simulink model "Sim_normboundsystem_iqctest"  (Simulink 7.3)
settings: Solver=ode45  StartTime=0.0  StopTime=10  RelTol=1e-3
settings Model: Creator=MD710  LastModifiedBy=MD710
settings DebuggingCC: SaveWithParameterizedLinksMsg=none  SolverPrmCheckMsg=none  MultiTaskDSMMsg=warning  MultiTaskCondExecSysMsg=none  FcnCallInpInsideContextMsg=Enable All  StrictBusMsg=None
settings HardwareCC: TargetHWDeviceType=32-bit Generic
settings RTWCC: IncludeERTFirstTime=on
settings GRTTargetCC: TargetFcnLib=ansi_tfl_tmw.mat

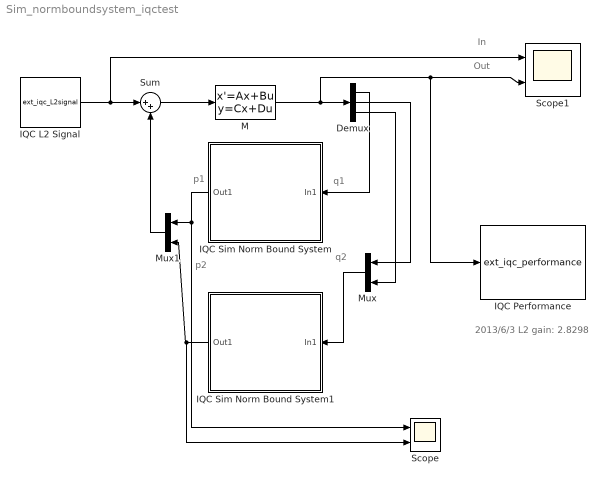
== system Sim_normboundsystem_iqctest ==
  note: p1
  note: q1
  note: q2
  note: p2
  note: 2013/6/3 L2 gain: 2.8298
  note: In
  note: Out
  Demux : Demux  Outputs=3
  IQC L2 Signal : M-S-Function  FunctionName=ext_iqc_L2signal  Parameters=sig_size,sam_time,sig_type,tru_time,sig_amp,sig_fre,user_cus  mask(IQC L2 signal(ver:0.1)){sig_size=2, sam_time=0, sig_type=Sine wave, tru_time=5, sig_amp=1, sig_fre=2, user_cus='2*exp(3*t)'}
      mask prompts: sig_size "Signal Dimension:(Default: 1)"; sam_time "Sample Time:(Default: 0)"; sig_type "Signal Type:"; tru_time "Truncation Time:"; sig_amp "Maximum Amplitude:"; sig_fre "Frequency:"; user_cus "Custom:"
      mask help:
      | Important:
      | In IQC procedure step (as commond iqc_gain_tbx, the task is get
      | L2 gain value), regardless of the user to choose which option (ex sine...),
      | here regarded as generalized L2 signal.
      mask StyleString: edit,edit,popup(Step|Square wave|Sine wave|Custom|Random|External),edit,edit,edit,edit
      mask CallbackString: ||iqc_block_cho(gcb,'L2signal_type')||||
      mask TabNameString: Main,Main,Simulation,Simulation,Simulation,Simulation,Simulation
      mask Display: plot(0:0.1:10,[sin(0:0.1:6.2) zeros(1,38)])
  IQC Performance : M-S-Function  FunctionName=ext_iqc_performance  Parameters=imp_met,save_lin_com,isiqcbode,fre_ran,uselmitool,lmi_par  mask(IQC Performance(ver:0.1)){imp_met=Calculation and Simulation, save_lin_com=off, isiqcbode=off, fre_ran='', uselmitool=lmilab, lmi_par=''}
      mask prompts: imp_met "Implementation Methods"; save_lin_com "Save the Linear File and Command File"; isiqcbode "Display IQC Bode Figure"; fre_ran "Frequency Range:(Default: empty)"; uselmitool "LMI Tool:"; lmi_par "Parameter:(if empty use define)"
      mask help:
      | Important:
      | In IQC toolbox calculate step (as commond iqc_gain_tbx, the task is get
      | L2 gain value), regardless of the user to connect any signal input(Even if
      | not a signal), here regarded as generalized L2 signal.
      |
      | Example 1: setlmioptions('',[0 200 0 0 777])
      | the block parameter is
      | LMI Tool: lmilab
      | Parameter:
      |        [0 200 0 0 777]
      |
      | Example 2: setlmioptions('yalmip','solver','sdpt3','verbose',1)
      | the block parameter is
      | LMI Tool: yalmip
      | Parameter:
      |        {'solver',sdpt3','verbose',1}
      mask Help:
      | <a href="matlab:doc abst_init_iqc;">abst_init_iqc</a>
      | <a href="matlab:doc setlmioptions;">setlmioptions</a>
      | <a href="matlab:doc iqc_gain_tbx;">iqc_gain_tbx</a>
      mask StyleString: popup(Calculation and Simulation|Only Calculation|Only Simulation),checkbox,checkbox,edit,popup(lmilab|yalmip),edit
      mask CallbackString: iqc_block_cho(gcb,'performance_imp')||iqc_block_cho(gcb,'performance_bodefre')|||
      mask TabNameString: Main,Main,Main,Main,LMI,LMI
      mask Display: fprintf('In -> Out \n performance \n L2 gain:\n%4.4f',2.8297);
  IQC Sim Norm Bound System : Subsystem  mask(IQC Sim Norm Bound System(ver:0.1)){sou_sys=Random, num_inp=1, num_out=1, num_sta=3, upp_bou=1, sam_tim=0, cus='1/(s+1)', var_nam='', iqc1=on, iqc1_pole=[4], iqc1_out='', iqc2=on, lis_rel='out==iqc_ltigain(in)', swsystemtype=0, A=0, B=0, C=0, D=0, newsam_tim=0}
      mask prompts: sou_sys "Source of the system:(Default: Random)"; num_inp "The Number of Input:(Default: 1)"; num_out "The Number of Output:(Default: 1)"; num_sta "The Number of States:(Default: 1)"; upp_bou "Upper Bound of the Hinf-Norm:(default: 1)"; sam_tim "Sample Time:(Default: 0)"; cus "Custom: (Default: '1/(s+1)' or '1/(z+0.5)')"; var_nam "Variable Name:(Default: empty)"; iqc1 "iqc_ltiunmod(Input,Pole,Number Output,Upper Bound)"; iqc1_pole "Pole:(Default: [1])"; iqc1_out "Output Variable:(Default: empty)"; iqc2 "Custom IQC"; lis_rel "List of IQC Relationships:"; newsam_tim "Mask Parameter 19:"
      mask init:
      | swsystemtype=1;
      | A=randn(num_sta);
      | B=randn(num_sta,num_inp);
      | C=randn(num_out,num_sta);
      | D=randn(num_out,num_inp);
      | switch sou_sys
      |     case 1
      |         if sam_tim==0
      |             newsam_tim=1;
      |             A=A-(1+max(real(eig(A))))*eye(num_sta);
      |             G=ss(A,B,C,D);
      |             normG=norm(G,inf);
      |             G=G*upp_bou*rand/normG;
      |         elseif sam_tim>0
      |             newsam_tim=sam_tim;
      |             swsystemtype=2;
      |             A=A-(1+max(real(eig(A))))*eye(num_sta);
      |             G=ss(A,B,C,D);
      |             normG=norm(G,inf);
      |             G=G*upp_bou*rand/normG;
      |             G=c2d(G,sam_tim);
      |         else
      |             error(['sampletime set error'])
      |         end
      |     case 2
      |         s=tf('s');
      |         newsam_tim=1;
      |         if sam_tim>0
      |             newsam_tim=sam_tim;
      |             swsystemtype=2;
      |             z=tf('z',sam_tim);
      |         end
      |         if ischar(cus)
      |             eval(['G=ss(',cus,');']);
      |         else
      |             G=ss(cus);
      |         end
      | end
      | A=G.a;
      | B=G.b;
      | C=G.c;
      | D=G.d;
      mask Help: <a href="matlab:doc iqc_ltiunmod;">iqc_ltiunmod</a>
      mask StyleString: popup(Random|Custom),edit,edit,edit,edit,edit,edit,edit,checkbox,edit,edit,checkbox,edit,edit,edit,edit,edit,edit,edit
      mask CallbackString: iqc_block_cho(gcb,'sim_normboundsys_sou')||||||||iqc_block_cho(gcb,'sim_normboundsys_iqc1')|||iqc_block_cho(gcb,'sim_normboundsys_iqc2')|||||||
      mask TabNameString: Simulink Parameters,Simulink Parameters,Simulink Parameters,Simulink Parameters,Simulink Parameters,Simulink Parameters,Simulink Parameters,Simulink Parameters,Procedure Parameters,Procedure Parameters,Procedure Parameters,Procedure Parameters,Procedure Parameters,Simulink Parameters,Simulink Parameters,Simulink Parameters,Simulink Parameters,Simulink Parameters,Simulink Parameters
      mask Display: disp('\fontsize{14}||\Delta|| < k', 'texmode','on');
  IQC Sim Norm Bound System1 : Subsystem  mask(IQC Sim Norm Bound System(ver:0.1)){sou_sys=Random, num_inp=2, num_out=1, num_sta=5, upp_bou=1, sam_tim=0, cus='1/(s+1)', var_nam='', iqc1=on, iqc1_pole=[4], iqc1_out='', iqc2=off, lis_rel='out==iqc_ltigain(in)', swsystemtype=0, A=0, B=0, C=0, D=0, newsam_tim=0}
      mask prompts: sou_sys "Source of the system:(Default: Random)"; num_inp "The Number of Input:(Default: 1)"; num_out "The Number of Output:(Default: 1)"; num_sta "The Number of States:(Default: 1)"; upp_bou "Upper Bound of the Hinf-Norm:(default: 1)"; sam_tim "Sample Time:(Default: 0)"; cus "Custom: (Default: '1/(s+1)' or '1/(z+0.5)')"; var_nam "Variable Name:(Default: empty)"; iqc1 "iqc_ltiunmod(Input,Pole,Number Output,Upper Bound)"; iqc1_pole "Pole:(Default: [1])"; iqc1_out "Output Variable:(Default: empty)"; iqc2 "Custom IQC"; lis_rel "List of IQC Relationships:"; newsam_tim "Mask Parameter 19:"
      mask init: same as Sim_normboundsystem_iqctest/IQC Sim Norm Bound System
      mask Help: <a href="matlab:doc iqc_ltiunmod;">iqc_ltiunmod</a>
      mask StyleString: popup(Random|Custom),edit,edit,edit,edit,edit,edit,edit,checkbox,edit,edit,checkbox,edit,edit,edit,edit,edit,edit,edit
      mask CallbackString: iqc_block_cho(gcb,'sim_normboundsys_sou')||||||||iqc_block_cho(gcb,'sim_normboundsys_iqc1')|||iqc_block_cho(gcb,'sim_normboundsys_iqc2')|||||||
      mask TabNameString: Simulink Parameters,Simulink Parameters,Simulink Parameters,Simulink Parameters,Simulink Parameters,Simulink Parameters,Simulink Parameters,Simulink Parameters,Procedure Parameters,Procedure Parameters,Procedure Parameters,Procedure Parameters,Procedure Parameters,Simulink Parameters,Simulink Parameters,Simulink Parameters,Simulink Parameters,Simulink Parameters,Simulink Parameters
      mask Display: disp('\fontsize{14}||\Delta|| < k', 'texmode','on');
  M : StateSpace  A=[-100 0 0 0;0 -80 0 0;0 0 -10 0;0 0 0 -8]  B=[8 0;8 0;2 0;0 2]  C=[-8.333 0 0 0;0 -6.667 0 0;0 0 3.333 2.667]  D=[0.6667 0;0.6667 0;0 0]
  Mux : Mux  Inputs=2
  Mux1 : Mux  Inputs=2
  Scope : Scope  NumInputPorts=2
      settings: YMin=-0.7~-0.2  YMax=0.5~0.25
  Scope1 : Scope  NumInputPorts=2
      settings: YMin=-5~-5  YMax=5~5
  Sum : Sum  Inputs=|++
  wires:
  IQC L2 Signal/1 -> Sum/1, Scope1/1
  Sum/1 -> M/1
  M/1 -> Demux/1, IQC Performance/1, Scope1/2
  Demux/1 -> IQC Sim Norm Bound System/1(In1)
  Demux/2 -> Mux/1
  Demux/3 -> Mux/2
  IQC Sim Norm Bound System1/1(Out1) -> Scope/2, Mux1/2
  Mux1/1 -> Sum/2
  IQC Sim Norm Bound System/1(Out1) -> Scope/1, Mux1/1
  Mux/1 -> IQC Sim Norm Bound System1/1(In1)

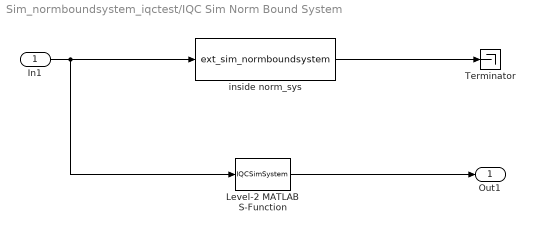
== system Sim_normboundsystem_iqctest/IQC Sim Norm Bound System ==
  In1 : Inport
  Level-2 MATLAB S-Function : M-S-Function  FunctionName=IQCSimSystem  Parameters=A,B,C,D,sam_tim
  Terminator : Terminator
  inside norm_sys : M-S-Function  FunctionName=ext_sim_normboundsystem  Parameters=sou_sys,num_inp,num_out,num_sta,upp_bou,sam_tim,cus,var_nam,iqc1,iqc1_pole,iqc1_out,iqc2,lis_rel,swsystemtype,A,B,C,D,
  Out1 : Outport
  wires:
  Level-2 MATLAB S-Function/1 -> Out1/1
  In1/1 -> inside norm_sys/1, Level-2 MATLAB S-Function/1
  inside norm_sys/1 -> Terminator/1

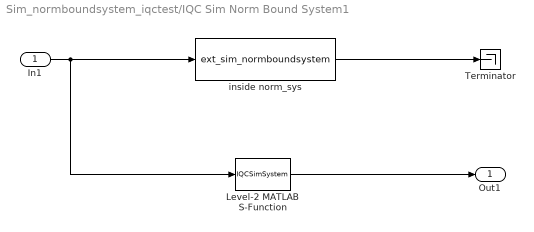
== system Sim_normboundsystem_iqctest/IQC Sim Norm Bound System1 ==
  In1 : Inport
  Level-2 MATLAB S-Function : M-S-Function  FunctionName=IQCSimSystem  Parameters=A,B,C,D,sam_tim
  Terminator : Terminator
  inside norm_sys : M-S-Function  FunctionName=ext_sim_normboundsystem  Parameters=sou_sys,num_inp,num_out,num_sta,upp_bou,sam_tim,cus,var_nam,iqc1,iqc1_pole,iqc1_out,iqc2,lis_rel,swsystemtype,A,B,C,D,
  Out1 : Outport
  wires:
  inside norm_sys/1 -> Terminator/1
  In1/1 -> Level-2 MATLAB S-Function/1, inside norm_sys/1
  Level-2 MATLAB S-Function/1 -> Out1/1
